simulink library "xrbsMath_r3"  (Simulink 5.0)
undefined symbols (not defined in the file or in its folder): num_width
libraries: xbsIndex_r3 x775, xrbsMath_r3 x16
(part 2 of 8)

== system xrbsMath_r3/CORDIC SQRT ==
  note: The CORDIC Square Root algorithm is implemented in 4 steps.
      |
      | Step 1: Co-ordinate Rotation.  The CORDIC algorithm converges only for positive values of x. If x < zero, the input data is
      | converted to a non-negative number. If x = 0, a zero detect flag is passed along. The Square Root circuit has been designed to
      | converge for all values of X, except for the most negative value .
      |
      | Step 2: Normalization.  The CORDIC algorithm converges only for 0.25 <= x < 1.0. During normalization, the input X is shifted to the
      | left till it has a 1 in the most significant bit after the signed bit. If the left shift resullted in an odd number of shift values, a right shift is
      | performed resulting in an even number of left shifts. The shift value is divided by 2 and passed on to the quadrant correct stage. The
      | square root is derived using the identity sqrt( w) = sqrt{ (w + 1/4)^2 - (w - 1/4)^2). Based on this identity the input w gets mapped to,
      | X = w + 0.25 and Y = w - 0.25.
      |
      | Step 3: Hyperbolic Rotations.  For sqrt(x^2 - y^2) calculation, the resulting vector is rotated through progressively smaller angles, such
      | that y goes to zero.
      |
      | Step 4: Co-ordinate Correction. If the input was negative and a left shift was applied to X, this step assigns the appropriate
      | sign to the resulting ratio and multiplies it with 2^(-shift). If the input was zero, the zero detect flag is used to set the output
      | to 0.
  x : Inport
  CORDIC Fine Angle PE : Subsystem  mask(CORDIC parallel PE){stages=stages, pe_nbits=norm_nbits+1, pe_binpt=norm_binpt, pipeline_x=pipeline, prev_stages=12, pipeline=[0  0  0  0  0  0  0  0  0  0  0  0]}
      mask prompts: stages "Number of Stages"; pe_nbits "Number of Bits"; pe_binpt "Binary Point Position"; pipeline_x "Pipeline Stage Value"; prev_stages "Previous Stages"; pipeline "Previous Pipeline Stage Value"
      mask init:
      | [bg,fg] = xlcmap('XBlock',0);
      | iPos = get_param(gcb,'Position');
      | iWidth=iPos(3)-iPos(1); iHeight=iPos(4)-iPos(2);
      | iCx=iWidth/2;
      | iCy=iHeight/2;
      | [logoX, logoY] = xlogo(iPos);
      | set_param(gcb,'LinkStatus', 'none');
      | sav_gcb=gcb;
      | stages = round(sum(abs(stages)));
      | if (stages == 0)
      | 	stages = prev_stages;
      | end
      | x = zeros(1,stages);
      | pipe_size = max(size(pipeline_x));
      | if pipe_size >= stages
      | 	x(1,1:stages) = pipeline_x(1,1:stages);
      | else
      | 	x(1,1:pipe_size) = pipeline_x(1,1:pipe_size);
      | end
      | 
      | if (stages ~=prev_stages)
      | 	pipeline = x;
      | 	a=find_system(sav_gcb, 'lookUnderMasks', 'all', 'FollowLinks','on','masktype', 'CORDIC iteration PE');
      | 	for i= 2:length(a)
      | 		for j=1:2
      | 		    delete_line(sav_gcb, ['CORDIC PE' int2str(i-1) '/' int2str(j)], ['CORDIC PE' int2str(i) '/' int2str(j)]);
      | 		end
      | 	end
      | 	delete_line(sav_gcb, ['CORDIC PE' int2str(length(a)) '/1'],'X/1');
      | 	delete_line(sav_gcb, ['CORDIC PE' int2str(length(a)) '/2'],'Terminator/1');
      | 	
      | 	for i=2:length(a)
      |       delete_block(a{i});
      | 	end
      | 	ite_stage=1;
      | 	repeat_stage=4;
      | 	dec_stage=0;
      | 	for i=2:stages
      |         ite_stage= i-dec_stage;
      | 		if(repeat_stage==ite_stage-1)
      |             ite_stage=ite_stage-1;
      | 			repeat_stage=repeat_stage*3+1;
      | 			dec_stage=dec_stage+1;
      | 		end
      |         add_block([sav_gcb '/CORDIC PE1'], [sav_gcb '/CORDIC PE' int2str(i)],'ii',int2str(ite_stage),'pipeline',['pipeline(1,' int2str(i) ')'],'position',[150+(i-1)*125, 70, 205+(i-1)*125, 130]);
      | 	end
      |     set_param([sav_gcb '/' 'X'], 'Position', [150+stages*125, 78, 180+stages*125, 92]);
      |     set_param([sav_gcb '/' 'Terminator'], 'Position', [210+stages*125, 107, 225+stages*125, 123]);
      |     for i= 2:stages
      | 		for j=1:2
      | 		    add_line(sav_gcb, ['CORDIC PE' int2str(i-1) '/' int2str(j)], ['CORDIC PE' int2str(i) '/' int2str(j)]);
      | 		end
      | 	end
      |     add_line(sav_gcb, ['CORDIC PE' int2str(stages) '/1'],'X/1');
      | 	add_line(sav_gcb, ['CORDIC PE' int2str(stages) '/2'],'Terminator/1');
      | 	find_system(sav_gcb, 'lookUnderMasks', 'all', 'FollowLinks', 'on', 'MaskType','Xilinx Slice Block');
      | 	set_param(sav_gcb, 'prev_stages',int2str(stages));
      | 	set_param(sav_gcb, 'pipeline', [ '[' int2str(x) ']']);
      | end
      | 
      | if (sum(pipeline~=x))
      | 	pipeline = x;
      | 	set_param(sav_gcb, 'pipeline', [ '[' int2str(x) ']']);
      | end
      mask Display:
      | patch([0 iWidth iWidth 0],[0 0 iHeight iHeight] , bg);
      | patch(logoX,logoY , fg);
      | port_label('input',1,'x');
      | port_label('input',2,'y');
      | port_label('input',3,'sgn(x)');
      | port_label('input',4,'shift');
      | port_label('input',5,'0_det');
      | port_label('output',1,'X');
      | port_label('output',2,'sgn(x)');
      | port_label('output',3,'shift');
      | port_label('output',4,'0_det');
      | plot([0 0 iWidth iWidth 0], [0 iHeight iHeight 0 0]);
  Quadrant Correct : Subsystem
      mask init:
      | [bg,fg] = xlcmap('XBlock',0);
      | iPos = get_param(gcb,'Position');
      | iWidth=iPos(3)-iPos(1); iHeight=iPos(4)-iPos(2);
      | iCx=iWidth/2;
      | iCy=iHeight/2;
      | [logoX, logoY] = xlogo(iPos);
      mask Display:
      | patch([0 iWidth iWidth 0],[0 0 iHeight iHeight] , bg);
      | patch(logoX,logoY , fg);
      | port_label('input',1,'X');
      | port_label('input',2,'sgn(x)');
      | port_label('input',3,'shift');
      | port_label('input',4,'0_det');
      | port_label('output',1,'X');
      | plot([0 0 iWidth iWidth 0], [0 iHeight iHeight 0 0]);
  Quadrant Map : Subsystem
      mask init:
      | [bg,fg] = xlcmap('XBlock',0);
      | iPos = get_param(gcb,'Position');
      | iWidth=iPos(3)-iPos(1); iHeight=iPos(4)-iPos(2);
      | iCx=iWidth/2;
      | iCy=iHeight/2;
      | [logoX, logoY] = xlogo(iPos);
      mask Display:
      | patch([0 iWidth iWidth 0],[0 0 iHeight iHeight] , bg);
      | patch(logoX,logoY , fg);
      | port_label('input',1,'x');
      | port_label('output',1,'X');
      | port_label('output',2,'Y');
      | port_label('output',3,'sgn(x)');
      | port_label('output',4,'shift');
      | port_label('output',5,'0_det');
      | plot([0 0 iWidth iWidth 0], [0 iHeight iHeight 0 0]);
  X : Outport
  wires:
  Quadrant Map/1(X) -> CORDIC Fine Angle PE/1(x)
  Quadrant Map/2(Y) -> CORDIC Fine Angle PE/2(y)
  Quadrant Correct/1(Z) -> X/1
  CORDIC Fine Angle PE/1(X) -> Quadrant Correct/1(X)
  x/1 -> Quadrant Map/1(x)
  Quadrant Map/3(sign(x)) -> CORDIC Fine Angle PE/3(sign)
  Quadrant Map/4(shift) -> CORDIC Fine Angle PE/4(shift)
  CORDIC Fine Angle PE/2(sign_dly) -> Quadrant Correct/2(sign_x)
  CORDIC Fine Angle PE/3(shift_dly) -> Quadrant Correct/3(shift)
  Quadrant Map/5(zero_detect) -> CORDIC Fine Angle PE/5(zero_detect)
  CORDIC Fine Angle PE/4(zero_detect_dly) -> Quadrant Correct/4(zero_detect)

== system xrbsMath_r3/CORDIC ATAN/CORDIC Fine Angle PE ==
  note: The fine angle rotation operation is performed iteratively in stages (0..stages-1).
      | The i-th PE rotates its input vector by an angle +/- atan(1/2^i), driving its input y coordinate towards zero.
  x : Inport
  y : Inport  Port=2
  z : Inport  Port=3
  CORDIC PE1 : Subsystem  mask(CORDIC iteration PE){ii=0, pe_nbits=pe_nbits, pe_binpt=pe_binpt, epsilon_k_fcn=atan, epsilon_k=, pipeline=pipeline(1,1)}
      mask prompts: ii "Iteration Index ii"; pe_nbits "Number of X,Y,Z Bits"; pe_binpt "X,Y,Z Binary Point Position"; epsilon_k_fcn "Epsilon_k Function"; pipeline "Pipeline Latency"
      mask init:
      | [bg,fg] = xlcmap('XBlock',0);
      | iPos = get_param(gcb,'Position');
      | iWidth=iPos(3)-iPos(1); iHeight=iPos(4)-iPos(2);
      | iCx=iWidth/2;
      | iCy=iHeight/2;
      | [logoX, logoY] = xlogo(iPos);
      | 
      | set_param(gcb, 'LinkStatus', 'none');
      | switch epsilon_k_fcn
      |   case 1
      |     epsilon_k = atan(1/2^ii);
      |   case 2
      |     epsilon_k = atanh(1/2^ii);
      | end
      mask StyleString: edit,edit,edit,popup(atan|atanh),edit,edit
      mask Display:
      | patch([0 iWidth iWidth 0],[0 0 iHeight iHeight] , bg);
      | patch(logoX,logoY , fg);
      | port_label('input',1,'x');
      | port_label('input',2,'y');
      | port_label('input',3,'z');
      | port_label('output',1,'X');
      | port_label('output',2,'Y');
      | port_label('output',3,'Z');
      | plot([0 0 iWidth iWidth 0], [0 iHeight iHeight 0 0]);
  CORDIC PE2 : Subsystem  mask(CORDIC iteration PE){ii=1, pe_nbits=pe_nbits, pe_binpt=pe_binpt, epsilon_k_fcn=atan, epsilon_k=, pipeline=pipeline(1,2)}
      mask prompts: ii "Iteration Index ii"; pe_nbits "Number of X,Y,Z Bits"; pe_binpt "X,Y,Z Binary Point Position"; epsilon_k_fcn "Epsilon_k Function"; pipeline "Pipeline Latency"
      mask init: same as xrbsMath_r3/CORDIC ATAN/CORDIC Fine Angle PE/CORDIC PE1
      mask StyleString: edit,edit,edit,popup(atan|atanh),edit,edit
      mask Display:
      | patch([0 iWidth iWidth 0],[0 0 iHeight iHeight] , bg);
      | patch(logoX,logoY , fg);
      | port_label('input',1,'x');
      | port_label('input',2,'y');
      | port_label('input',3,'z');
      | port_label('output',1,'X');
      | port_label('output',2,'Y');
      | port_label('output',3,'Z');
      | plot([0 0 iWidth iWidth 0], [0 iHeight iHeight 0 0]);
  CORDIC PE3 : Subsystem  mask(CORDIC iteration PE){ii=2, pe_nbits=pe_nbits, pe_binpt=pe_binpt, epsilon_k_fcn=atan, epsilon_k=, pipeline=pipeline(1,3)}
      mask prompts: ii "Iteration Index ii"; pe_nbits "Number of X,Y,Z Bits"; pe_binpt "X,Y,Z Binary Point Position"; epsilon_k_fcn "Epsilon_k Function"; pipeline "Pipeline Latency"
      mask init: same as xrbsMath_r3/CORDIC ATAN/CORDIC Fine Angle PE/CORDIC PE1
      mask StyleString: edit,edit,edit,popup(atan|atanh),edit,edit
      mask Display:
      | patch([0 iWidth iWidth 0],[0 0 iHeight iHeight] , bg);
      | patch(logoX,logoY , fg);
      | port_label('input',1,'x');
      | port_label('input',2,'y');
      | port_label('input',3,'z');
      | port_label('output',1,'X');
      | port_label('output',2,'Y');
      | port_label('output',3,'Z');
      | plot([0 0 iWidth iWidth 0], [0 iHeight iHeight 0 0]);
  CORDIC PE4 : Subsystem  mask(CORDIC iteration PE){ii=3, pe_nbits=pe_nbits, pe_binpt=pe_binpt, epsilon_k_fcn=atan, epsilon_k=, pipeline=pipeline(1,4)}
      mask prompts: ii "Iteration Index ii"; pe_nbits "Number of X,Y,Z Bits"; pe_binpt "X,Y,Z Binary Point Position"; epsilon_k_fcn "Epsilon_k Function"; pipeline "Pipeline Latency"
      mask init: same as xrbsMath_r3/CORDIC ATAN/CORDIC Fine Angle PE/CORDIC PE1
      mask StyleString: edit,edit,edit,popup(atan|atanh),edit,edit
      mask Display:
      | patch([0 iWidth iWidth 0],[0 0 iHeight iHeight] , bg);
      | patch(logoX,logoY , fg);
      | port_label('input',1,'x');
      | port_label('input',2,'y');
      | port_label('input',3,'z');
      | port_label('output',1,'X');
      | port_label('output',2,'Y');
      | port_label('output',3,'Z');
      | plot([0 0 iWidth iWidth 0], [0 iHeight iHeight 0 0]);
  CORDIC PE5 : Subsystem  mask(CORDIC iteration PE){ii=4, pe_nbits=pe_nbits, pe_binpt=pe_binpt, epsilon_k_fcn=atan, epsilon_k=, pipeline=pipeline(1,5)}
      mask prompts: ii "Iteration Index ii"; pe_nbits "Number of X,Y,Z Bits"; pe_binpt "X,Y,Z Binary Point Position"; epsilon_k_fcn "Epsilon_k Function"; pipeline "Pipeline Latency"
      mask init: same as xrbsMath_r3/CORDIC ATAN/CORDIC Fine Angle PE/CORDIC PE1
      mask StyleString: edit,edit,edit,popup(atan|atanh),edit,edit
      mask Display:
      | patch([0 iWidth iWidth 0],[0 0 iHeight iHeight] , bg);
      | patch(logoX,logoY , fg);
      | port_label('input',1,'x');
      | port_label('input',2,'y');
      | port_label('input',3,'z');
      | port_label('output',1,'X');
      | port_label('output',2,'Y');
      | port_label('output',3,'Z');
      | plot([0 0 iWidth iWidth 0], [0 iHeight iHeight 0 0]);
  CORDIC PE6 : Subsystem  mask(CORDIC iteration PE){ii=5, pe_nbits=pe_nbits, pe_binpt=pe_binpt, epsilon_k_fcn=atan, epsilon_k=, pipeline=pipeline(1,6)}
      mask prompts: ii "Iteration Index ii"; pe_nbits "Number of X,Y,Z Bits"; pe_binpt "X,Y,Z Binary Point Position"; epsilon_k_fcn "Epsilon_k Function"; pipeline "Pipeline Latency"
      mask init: same as xrbsMath_r3/CORDIC ATAN/CORDIC Fine Angle PE/CORDIC PE1
      mask StyleString: edit,edit,edit,popup(atan|atanh),edit,edit
      mask Display:
      | patch([0 iWidth iWidth 0],[0 0 iHeight iHeight] , bg);
      | patch(logoX,logoY , fg);
      | port_label('input',1,'x');
      | port_label('input',2,'y');
      | port_label('input',3,'z');
      | port_label('output',1,'X');
      | port_label('output',2,'Y');
      | port_label('output',3,'Z');
      | plot([0 0 iWidth iWidth 0], [0 iHeight iHeight 0 0]);
  CORDIC PE7 : Subsystem  mask(CORDIC iteration PE){ii=6, pe_nbits=pe_nbits, pe_binpt=pe_binpt, epsilon_k_fcn=atan, epsilon_k=, pipeline=pipeline(1,7)}
      mask prompts: ii "Iteration Index ii"; pe_nbits "Number of X,Y,Z Bits"; pe_binpt "X,Y,Z Binary Point Position"; epsilon_k_fcn "Epsilon_k Function"; pipeline "Pipeline Latency"
      mask init: same as xrbsMath_r3/CORDIC ATAN/CORDIC Fine Angle PE/CORDIC PE1
      mask StyleString: edit,edit,edit,popup(atan|atanh),edit,edit
      mask Display:
      | patch([0 iWidth iWidth 0],[0 0 iHeight iHeight] , bg);
      | patch(logoX,logoY , fg);
      | port_label('input',1,'x');
      | port_label('input',2,'y');
      | port_label('input',3,'z');
      | port_label('output',1,'X');
      | port_label('output',2,'Y');
      | port_label('output',3,'Z');
      | plot([0 0 iWidth iWidth 0], [0 iHeight iHeight 0 0]);
  CORDIC PE8 : Subsystem  mask(CORDIC iteration PE){ii=7, pe_nbits=pe_nbits, pe_binpt=pe_binpt, epsilon_k_fcn=atan, epsilon_k=, pipeline=pipeline(1,8)}
      mask prompts: ii "Iteration Index ii"; pe_nbits "Number of X,Y,Z Bits"; pe_binpt "X,Y,Z Binary Point Position"; epsilon_k_fcn "Epsilon_k Function"; pipeline "Pipeline Latency"
      mask init: same as xrbsMath_r3/CORDIC ATAN/CORDIC Fine Angle PE/CORDIC PE1
      mask StyleString: edit,edit,edit,popup(atan|atanh),edit,edit
      mask Display:
      | patch([0 iWidth iWidth 0],[0 0 iHeight iHeight] , bg);
      | patch(logoX,logoY , fg);
      | port_label('input',1,'x');
      | port_label('input',2,'y');
      | port_label('input',3,'z');
      | port_label('output',1,'X');
      | port_label('output',2,'Y');
      | port_label('output',3,'Z');
      | plot([0 0 iWidth iWidth 0], [0 iHeight iHeight 0 0]);
  Terminator : Terminator
  X : Outport
  Z : Outport  Port=2
  wires:
  CORDIC PE1/1(X) -> CORDIC PE2/1(x)
  CORDIC PE1/2(Y) -> CORDIC PE2/2(y)
  CORDIC PE1/3(Z) -> CORDIC PE2/3(z)
  CORDIC PE2/1(X) -> CORDIC PE3/1(x)
  CORDIC PE2/2(Y) -> CORDIC PE3/2(y)
  CORDIC PE2/3(Z) -> CORDIC PE3/3(z)
  CORDIC PE3/1(X) -> CORDIC PE4/1(x)
  CORDIC PE3/2(Y) -> CORDIC PE4/2(y)
  CORDIC PE3/3(Z) -> CORDIC PE4/3(z)
  CORDIC PE4/1(X) -> CORDIC PE5/1(x)
  CORDIC PE4/2(Y) -> CORDIC PE5/2(y)
  CORDIC PE4/3(Z) -> CORDIC PE5/3(z)
  CORDIC PE5/1(X) -> CORDIC PE6/1(x)
  CORDIC PE5/2(Y) -> CORDIC PE6/2(y)
  CORDIC PE5/3(Z) -> CORDIC PE6/3(z)
  CORDIC PE6/1(X) -> CORDIC PE7/1(x)
  CORDIC PE6/2(Y) -> CORDIC PE7/2(y)
  CORDIC PE6/3(Z) -> CORDIC PE7/3(z)
  CORDIC PE7/1(X) -> CORDIC PE8/1(x)
  CORDIC PE7/2(Y) -> CORDIC PE8/2(y)
  CORDIC PE7/3(Z) -> CORDIC PE8/3(z)
  x/1 -> CORDIC PE1/1(x)
  y/1 -> CORDIC PE1/2(y)
  z/1 -> CORDIC PE1/3(z)
  CORDIC PE8/1(X) -> X/1
  CORDIC PE8/2(Y) -> Terminator/1
  CORDIC PE8/3(Z) -> Z/1

== system xrbsMath_r3/CORDIC ATAN/Quadrant Correct ==
  note: The  CORDIC algorithm coverges for angles between  -pi/2 to +pi/2. The Quadrant Correct subsystem reflects
      | the angle back to the 2nd and 3rd quadrant from the 1st and 4th quadarnt if reflection was applied during the
      | quadarnt map stage. Reflection is applied by subtracting the output angle by pi if the original vector was in the
      | 2nd quadrant and -p if it was in the 3rd quadrant.
  Z IN : Inport
  PI_ addsub : Inport  Port=2
  Z MUX SEL : Inport  Port=3
  +PI : xbsIndex_r3/Constant  const=pi  arith_type="Signed  (2's comp)"  n_bits=pe_nbits  bin_pt=pe_binpt  explicit_period=off  period=1  dbl_ovrd=off
  -PI : xbsIndex_r3/Constant  const=-pi  arith_type="Signed  (2's comp)"  n_bits=pe_nbits  bin_pt=pe_binpt  explicit_period=off  period=1  dbl_ovrd=off
  AddSub : xbsIndex_r3/AddSub  mode=Subtraction  precision=User Defined  arith_type="Signed  (2's comp)"  n_bits=pe_nbits  bin_pt=pe_binpt  quantization=Truncate  overflow=Wrap  latency=0  explicit_period=off  period=1  en=off  dbl_ovrd=off  use_core=on  gen_core=on  pipeline=off  use_rpm=off
      settings: xl_area=[0, 0, 0, 0, 0, 0, 0]
  Convert : xbsIndex_r3/Convert  arith_type=Boolean  n_bits=8  bin_pt=6  quantization=Truncate  overflow=Wrap  latency=0  explicit_period=off  period=1  dbl_ovrd=off  inserted_by_tool=off
      settings: xl_area=[0, 0, 0, 0, 0, 0, 0]
  Mux : xbsIndex_r3/Mux  inputs=2  precision=Full  arith_type="Signed  (2's comp)"  n_bits=8  bin_pt=2  quantization=Truncate  overflow=Wrap  latency=1  mux_type=off  explicit_period=off  period=1  en=off  dbl_ovrd=off  gen_core=on  use_rpm=off
      settings: xl_area=[0, 0, 0, 0, 0, 0, 0]
  Mux1 : xbsIndex_r3/Mux  inputs=2  precision=Full  arith_type="Signed  (2's comp)"  n_bits=8  bin_pt=2  quantization=Truncate  overflow=Wrap  latency=0  mux_type=off  explicit_period=off  period=1  en=off  dbl_ovrd=off  gen_core=on  use_rpm=off
      settings: xl_area=[0, 0, 0, 0, 0, 0, 0]
  Z : Outport
  wires:
  -PI/1 -> Mux1/3
  +PI/1 -> Mux1/2
  Mux1/1 -> AddSub/1
  Convert/1 -> Mux1/1
  Z IN/1 -> Mux/2, AddSub/2
  Mux/1 -> Z/1
  AddSub/1 -> Mux/3
  Z MUX SEL/1 -> Mux/1
  PI_ addsub/1 -> Convert/1

== system xrbsMath_r3/CORDIC ATAN/Quadrant Map ==
  note: The  CORDIC algorithm converges for angles between  -pi/2 to +pi/2. The Quadrant Map subsystem always maps the
      | absolute value for x-axis. This reflects the input vector from the 2nd and 3rd quadrant to the 1st and 4th quadrant, resp.
  x : Inport
  y : Inport  Port=2
  Delay3 : xbsIndex_r3/Delay  latency=2  explicit_period=off  period=1  en=off  accept_only_valid=off  init_zero=on  dbl_ovrd=off
      settings: xl_area=[0, 0, 0, 0, 0, 0, 0]
  Delay4 : xbsIndex_r3/Delay  latency=1  explicit_period=off  period=1  en=off  accept_only_valid=off  init_zero=on  dbl_ovrd=off
      settings: xl_area=[0, 0, 0, 0, 0, 0, 0]
  Mux : xbsIndex_r3/Mux  inputs=2  precision=User Defined  arith_type="Signed  (2's comp)"  n_bits=pe_nbits  bin_pt=pe_binpt  quantization=Truncate  overflow=Wrap  latency=1  mux_type=off  explicit_period=off  period=1  en=off  dbl_ovrd=off  gen_core=on  use_rpm=off
      settings: xl_area=[0, 0, 0, 0, 0, 0, 0]
  Negate1 : xbsIndex_r3/Negate  precision=User Defined  arith_type="Signed  (2's comp)"  n_bits=pe_nbits  bin_pt=pe_binpt  quantization=Truncate  overflow=Wrap  latency=0  explicit_period=off  period=1  en=off  dbl_ovrd=off  use_core=on  gen_core=on  use_rpm=off
      settings: xl_area=[0, 0, 0, 0, 0, 0, 0]
  sgn(x) : xbsIndex_r3/Slice  mode=Upper Bit Location + Width  nbits=1  bit1=0  base1=MSB of Input  bit0=0  base0=LSB of Input  boolean_output=off  explicit_period=off  period=1  dbl_ovrd=off
  sgn(y) : xbsIndex_r3/Slice  mode=Upper Bit Location + Width  nbits=1  bit1=0  base1=MSB of Input  bit0=0  base0=LSB of Input  boolean_output=off  explicit_period=off  period=1  dbl_ovrd=off
  X : Outport
  Y : Outport  Port=2
  sign(y) : Outport  Port=3
  sign(x) : Outport  Port=4
  wires:
  Delay3/1 -> Y/1, sgn(y)/1
  Negate1/1 -> Mux/3
  Mux/1 -> X/1
  y/1 -> Delay3/1
  x/1 -> Delay4/1
  sgn(x)/1 -> Mux/1, sign(x)/1
  sgn(y)/1 -> sign(y)/1
  Delay4/1 -> sgn(x)/1, Negate1/1, Mux/2

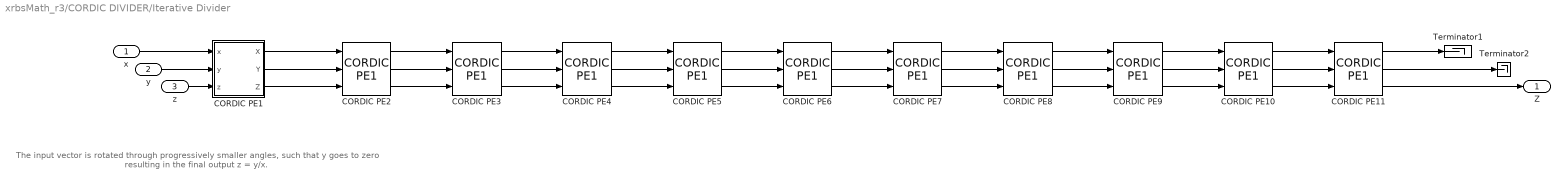
== system xrbsMath_r3/CORDIC DIVIDER/Iterative Divider ==
  note: The input vector is rotated through progressively smaller angles, such that y goes
      | to zero resulting in the final output z = y/x.
  x : Inport
  y : Inport  Port=2
  z : Inport  Port=3
  CORDIC PE1 : Subsystem  mask(CORDIC iteration Divider){ii=0, pe_nbits=num_width, pe_binpt=num_binpt, pipeline=pipeline(1,1), stages=stages}
      mask prompts: ii "Iteration Index ii"; pe_nbits "Number of X,Y,Z Bits"; pe_binpt "X,Y,Z Binary Point Position"; pipeline "Pipeline Latency"
      mask init:
      | [bg,fg] = xlcmap('XBlock',0);
      | iPos = get_param(gcb,'Position');
      | iWidth=iPos(3)-iPos(1); iHeight=iPos(4)-iPos(2);
      | iCx=iWidth/2;
      | iCy=iHeight/2;
      | [logoX, logoY] = xlogo(iPos);
      mask Display:
      | patch([0 iWidth iWidth 0],[0 0 iHeight iHeight] , bg);
      | patch(logoX,logoY , fg);
      | port_label('input',1,'x');
      | port_label('input',2,'y');
      | port_label('input',3,'z');
      | port_label('output',1,'X');
      | port_label('output',2,'Y');
      | port_label('output',3,'Z');
      | plot([0 0 iWidth iWidth 0], [0 iHeight iHeight 0 0]);
  CORDIC PE10 : xrbsMath_r3/CORDIC DIVIDER/Iterative Divider/CORDIC PE1  ii=9  pe_nbits=num_width  pe_binpt=num_binpt  pipeline=pipeline(1,10)  stages=stages
  CORDIC PE11 : xrbsMath_r3/CORDIC DIVIDER/Iterative Divider/CORDIC PE1  ii=10  pe_nbits=num_width  pe_binpt=num_binpt  pipeline=pipeline(1,11)  stages=stages
  CORDIC PE2 : xrbsMath_r3/CORDIC DIVIDER/Iterative Divider/CORDIC PE1  ii=1  pe_nbits=num_width  pe_binpt=num_binpt  pipeline=pipeline(1,2)  stages=stages
  CORDIC PE3 : xrbsMath_r3/CORDIC DIVIDER/Iterative Divider/CORDIC PE1  ii=2  pe_nbits=num_width  pe_binpt=num_binpt  pipeline=pipeline(1,3)  stages=stages
  CORDIC PE4 : xrbsMath_r3/CORDIC DIVIDER/Iterative Divider/CORDIC PE1  ii=3  pe_nbits=num_width  pe_binpt=num_binpt  pipeline=pipeline(1,4)  stages=stages
  CORDIC PE5 : xrbsMath_r3/CORDIC DIVIDER/Iterative Divider/CORDIC PE1  ii=4  pe_nbits=num_width  pe_binpt=num_binpt  pipeline=pipeline(1,5)  stages=stages
  CORDIC PE6 : xrbsMath_r3/CORDIC DIVIDER/Iterative Divider/CORDIC PE1  ii=5  pe_nbits=num_width  pe_binpt=num_binpt  pipeline=pipeline(1,6)  stages=stages
  CORDIC PE7 : xrbsMath_r3/CORDIC DIVIDER/Iterative Divider/CORDIC PE1  ii=6  pe_nbits=num_width  pe_binpt=num_binpt  pipeline=pipeline(1,7)  stages=stages
  CORDIC PE8 : xrbsMath_r3/CORDIC DIVIDER/Iterative Divider/CORDIC PE1  ii=7  pe_nbits=num_width  pe_binpt=num_binpt  pipeline=pipeline(1,8)  stages=stages
  CORDIC PE9 : xrbsMath_r3/CORDIC DIVIDER/Iterative Divider/CORDIC PE1  ii=8  pe_nbits=num_width  pe_binpt=num_binpt  pipeline=pipeline(1,9)  stages=stages
  Terminator1 : Terminator
  Terminator2 : Terminator
  Z : Outport
  wires:
  z/1 -> CORDIC PE1/3(z)
  y/1 -> CORDIC PE1/2(y)
  x/1 -> CORDIC PE1/1(x)
  CORDIC PE1/1(X) -> CORDIC PE2/1
  CORDIC PE1/2(Y) -> CORDIC PE2/2
  CORDIC PE1/3(Z) -> CORDIC PE2/3
  CORDIC PE2/1 -> CORDIC PE3/1
  CORDIC PE2/2 -> CORDIC PE3/2
  CORDIC PE2/3 -> CORDIC PE3/3
  CORDIC PE3/1 -> CORDIC PE4/1
  CORDIC PE3/2 -> CORDIC PE4/2
  CORDIC PE3/3 -> CORDIC PE4/3
  CORDIC PE4/1 -> CORDIC PE5/1
  CORDIC PE4/2 -> CORDIC PE5/2
  CORDIC PE4/3 -> CORDIC PE5/3
  CORDIC PE5/1 -> CORDIC PE6/1
  CORDIC PE5/2 -> CORDIC PE6/2
  CORDIC PE5/3 -> CORDIC PE6/3
  CORDIC PE6/1 -> CORDIC PE7/1
  CORDIC PE6/2 -> CORDIC PE7/2
  CORDIC PE6/3 -> CORDIC PE7/3
  CORDIC PE7/1 -> CORDIC PE8/1
  CORDIC PE7/2 -> CORDIC PE8/2
  CORDIC PE7/3 -> CORDIC PE8/3
  CORDIC PE8/1 -> CORDIC PE9/1
  CORDIC PE8/2 -> CORDIC PE9/2
  CORDIC PE8/3 -> CORDIC PE9/3
  CORDIC PE9/1 -> CORDIC PE10/1
  CORDIC PE9/2 -> CORDIC PE10/2
  CORDIC PE9/3 -> CORDIC PE10/3
  CORDIC PE10/1 -> CORDIC PE11/1
  CORDIC PE10/2 -> CORDIC PE11/2
  CORDIC PE10/3 -> CORDIC PE11/3
  CORDIC PE11/1 -> Terminator1/1
  CORDIC PE11/2 -> Terminator2/1
  CORDIC PE11/3 -> Z/1

== system xrbsMath_r3/CORDIC DIVIDER/Quadrant Correct ==
  note: Co-ordinate Correction. If the axis was rotated Step 1 and a relative shift was applied to Y over X, this step assigns the appropriate
      | sign to the resulting ratio and multiplies it with 2^(relative_shift of Y over X).
  z : Inport
  sign : Inport  Port=2
  norm : Inport  Port=3
  Mult : xbsIndex_r3/Mult  precision=Full  arith_type="Signed  (2's comp)"  n_bits=8  bin_pt=2  quantization=Truncate  overflow=Wrap  mult_type=Parallel  use_embedded=on  pipeline=on  latency=3  explicit_period=off  period=1  en=off  dbl_ovrd=off  oversample=2  use_rpm=off  placement_style=Rectangular Shape  gen_core=on
      settings: xl_area=[32 64 0 0 0 1 0]
  Mux : xbsIndex_r3/Mux  inputs=2  precision=Full  arith_type=Unsigned  n_bits=num_width-1  bin_pt=num_binpt  quantization=Truncate  overflow=Wrap  latency=0  mux_type=off  explicit_period=off  period=1  en=off  dbl_ovrd=off  use_rpm=off  gen_core=on
      settings: xl_area=[8 0 0 16 0 0 0]
  Negate : xbsIndex_r3/Negate  precision=User Defined  arith_type="Signed  (2's comp)"  n_bits=num_width  bin_pt=num_binpt  quantization=Truncate  overflow=Wrap  latency=0  explicit_period=off  period=1  en=off  dbl_ovrd=off  use_core=on  use_rpm=off  gen_core=on
      settings: xl_area=[8 0 0 16 0 0 0]
  ROM : xbsIndex_r3/ROM  depth=2^ceil(log2(num_width))  initVector=2.^(0:(2^ceil(log2(num_width))-1))  arith_type=Unsigned  n_bits=num_width  bin_pt=0  latency=0  distributed_mem=on  init_zero=on  explicit_period=off  period=1  rst=off  init_reg=0  en=off  dbl_ovrd=off  use_rpm=off  gen_core=on
      settings: xl_area=[8 0 0 16 0 0 0]
  Z : Outport
  wires:
  ROM/1 -> Mult/2
  Mult/1 -> Z/1
  norm/1 -> ROM/1
  Negate/1 -> Mux/3
  z/1 -> Negate/1, Mux/2
  sign/1 -> Mux/1
  Mux/1 -> Mult/1

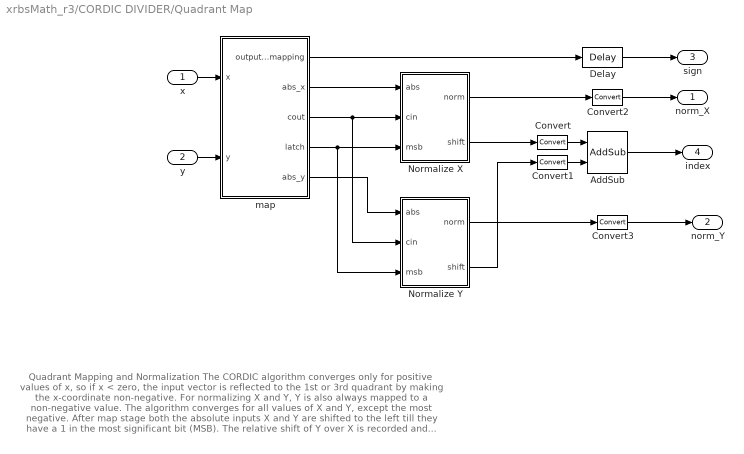
== system xrbsMath_r3/CORDIC DIVIDER/Quadrant Map ==
  note: Quadrant Mapping and Normalization
      |
      | The CORDIC algorithm converges only for positive values of x, so if x < zero, the input vector is reflected
      | to the 1st or 3rd quadrant by making the x-coordinate non-negative. For normalizing X and Y, Y is also
      | always mapped to a non-negative value. The algorithm converges for all values of X and Y, except the most negative.
      | After map stage both the absolute inputs X and Y are shifted to the left till they have a 1 in the most significant
      | bit (MSB). The relative shift of Y over X is recorded and passed on to the Quadrant Correct Stage.
  x : Inport
  y : Inport  Port=2
  AddSub : xbsIndex_r3/AddSub  mode=Subtraction  precision=User Defined  arith_type=Unsigned  n_bits=ceil(log2(num_width))  bin_pt=0  quantization=Truncate  overflow=Wrap  latency=0  explicit_period=off  period=1  en=off  dbl_ovrd=off  use_core=on  pipeline=off  use_rpm=off  gen_core=on
      settings: xl_area=[2 0 0 4 0 0 0]
  Convert : xbsIndex_r3/Convert  arith_type=Unsigned  n_bits=ceil(log2(num_width+1))  bin_pt=0  quantization=Truncate  overflow=Wrap  latency=0  explicit_period=off  period=1  dbl_ovrd=off  inserted_by_tool=off
      settings: xl_area=[0 0 0 0 0 0 0]
  Convert1 : xbsIndex_r3/Convert  arith_type=Unsigned  n_bits=ceil(log2(num_width+1))  bin_pt=0  quantization=Truncate  overflow=Wrap  latency=0  explicit_period=off  period=1  dbl_ovrd=off  inserted_by_tool=off
      settings: xl_area=[0 0 0 0 0 0 0]
  Convert2 : xbsIndex_r3/Convert  arith_type="Signed  (2's comp)"  n_bits=num_width  bin_pt=num_binpt  quantization=Truncate  overflow=Wrap  latency=0  explicit_period=off  period=1  dbl_ovrd=off  inserted_by_tool=off
      settings: xl_area=[0 0 0 0 0 0 0]
  Convert3 : xbsIndex_r3/Convert  arith_type="Signed  (2's comp)"  n_bits=num_width  bin_pt=num_binpt  quantization=Truncate  overflow=Wrap  latency=0  explicit_period=off  period=1  dbl_ovrd=off  inserted_by_tool=off
      settings: xl_area=[0 0 0 0 0 0 0]
  Delay : xbsIndex_r3/Delay  latency=num_width  reg_retiming=off  explicit_period=off  period=1  en=off  accept_only_valid=off  init_zero=on  dbl_ovrd=off
      settings: xl_area=[1 1 0 1 0 0 0]
  Normalize X : Subsystem  mask(Normalize X){num_bits=num_width-1, bin_point=num_binpt, prev_bits=15}
      mask prompts: num_bits "Number of bits"; bin_point "Binary Point Position"; prev_bits "Previous Number of bits"
      mask init:
      | [bg,fg] = xlcmap('XBlock',0);
      | iPos = get_param(gcb,'Position');
      | iWidth=iPos(3)-iPos(1); iHeight=iPos(4)-iPos(2);
      | iCx=iWidth/2;
      | iCy=iHeight/2;
      | [logoX, logoY] = xlogo(iPos);
      mask Display:
      | patch([0 iWidth iWidth 0],[0 0 iHeight iHeight] , bg);
      | patch(logoX,logoY , fg);
      | port_label('input',1,'abs');
      | port_label('input',2,'cin');
      | port_label('input',3,'msb');
      | port_label('output',1,'norm');
      | port_label('output',2,'shift');
      | plot([0 0 iWidth iWidth 0], [0 iHeight iHeight 0 0]);
  Normalize Y : Subsystem  mask(Normalize Y){num_bits=num_width-1, bin_point=num_binpt, prev_bits=15}
      mask prompts: num_bits "Number of bits"; bin_point "Binary Point Position"; prev_bits "Previous Number of bits"
      mask init:
      | [bg,fg] = xlcmap('XBlock',0);
      | iPos = get_param(gcb,'Position');
      | iWidth=iPos(3)-iPos(1); iHeight=iPos(4)-iPos(2);
      | iCx=iWidth/2;
      | iCy=iHeight/2;
      | [logoX, logoY] = xlogo(iPos);
      mask Display:
      | patch([0 iWidth iWidth 0],[0 0 iHeight iHeight] , bg);
      | patch(logoX,logoY , fg);
      | port_label('input',1,'abs');
      | port_label('input',2,'cin');
      | port_label('input',3,'msb');
      | port_label('output',1,'norm');
      | port_label('output',2,'shift');
      | plot([0 0 iWidth iWidth 0], [0 iHeight iHeight 0 0]);
  map : Subsystem
  norm_X : Outport
  norm_Y : Outport  Port=2
  sign : Outport  Port=3
  index : Outport  Port=4
  wires:
  map/1(output_mapping) -> Delay/1
  x/1 -> map/1(x)
  Normalize X/2(shift) -> Convert/1
  Normalize X/1(norm) -> Convert2/1
  Normalize Y/2(shift) -> Convert1/1
  Normalize Y/1(norm) -> Convert3/1
  y/1 -> map/2(y)
  map/2(abs_x) -> Normalize X/1(abs)
  map/3(cout) -> Normalize X/2(cin), Normalize Y/2(cin)
  map/4(latch) -> Normalize X/3(msb), Normalize Y/3(msb)
  map/5(abs_y) -> Normalize Y/1(abs)
  Convert/1 -> AddSub/1
  Convert1/1 -> AddSub/2
  AddSub/1 -> index/1
  Delay/1 -> sign/1
  Convert2/1 -> norm_X/1
  Convert3/1 -> norm_Y/1

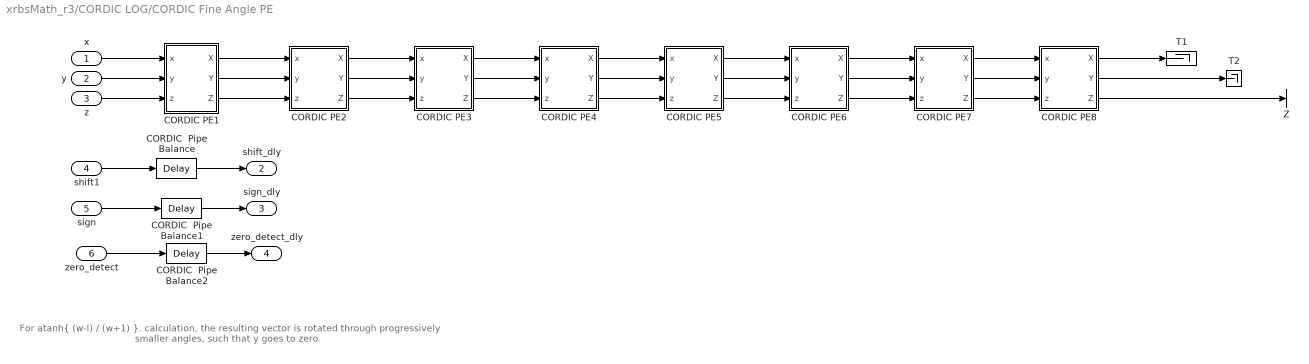
== system xrbsMath_r3/CORDIC LOG/CORDIC Fine Angle PE ==
  note: For atanh{ (w-l) / (w+1) }. calculation, the resulting vector is rotated through progressively smaller
      | angles, such that y goes to zero.
  x : Inport
  y : Inport  Port=2
  z : Inport  Port=3
  shift1 : Inport  Port=4
  sign : Inport  Port=5
  zero_detect : Inport  Port=6
  CORDIC  Pipe Balance : xbsIndex_r3/Delay  latency=sum(pipeline)  reg_retiming=off  explicit_period=off  period=1  en=off  accept_only_valid=off  init_zero=on  dbl_ovrd=off
      settings: xl_area=[1 1 0 1 0 0 0]
  CORDIC  Pipe Balance1 : xbsIndex_r3/Delay  latency=sum(pipeline)  reg_retiming=off  explicit_period=off  period=1  en=off  accept_only_valid=off  init_zero=on  dbl_ovrd=off
      settings: xl_area=[2 3 0 3 0 0 0]
  CORDIC  Pipe Balance2 : xbsIndex_r3/Delay  latency=sum(pipeline)  reg_retiming=off  explicit_period=off  period=1  en=off  accept_only_valid=off  init_zero=on  dbl_ovrd=off
      settings: xl_area=[1 1 0 1 0 0 0]
  CORDIC PE1 : Subsystem  mask(CORDIC iteration PE){ii=1, pe_nbits=pe_nbits, pe_binpt=pe_binpt, pipeline=pipeline(1,1)}
      mask prompts: ii "Iteration Index ii"; pe_nbits "Number of X,Y,Z Bits"; pe_binpt "X,Y,Z Binary Point Position"; pipeline "Pipeline Latency"
      mask init:
      | [bg,fg] = xlcmap('XBlock',0);
      | iPos = get_param(gcb,'Position');
      | iWidth=iPos(3)-iPos(1); iHeight=iPos(4)-iPos(2);
      | iCx=iWidth/2;
      | iCy=iHeight/2;
      | [logoX, logoY] = xlogo(iPos);
      | 
      | set_param(gcb, 'LinkStatus', 'none');
      mask Display:
      | patch([0 iWidth iWidth 0],[0 0 iHeight iHeight] , bg);
      | patch(logoX,logoY , fg);
      | port_label('input',1,'x');
      | port_label('input',2,'y');
      | port_label('input',3,'z');
      | port_label('output',1,'X');
      | port_label('output',2,'Y');
      | port_label('output',3,'Z');
      | plot([0 0 iWidth iWidth 0], [0 iHeight iHeight 0 0]);
  CORDIC PE2 : Subsystem  mask(CORDIC iteration PE){ii=2, pe_nbits=pe_nbits, pe_binpt=pe_binpt, pipeline=pipeline(1,2)}
      mask prompts: ii "Iteration Index ii"; pe_nbits "Number of X,Y,Z Bits"; pe_binpt "X,Y,Z Binary Point Position"; pipeline "Pipeline Latency"
      mask init: same as xrbsMath_r3/CORDIC LOG/CORDIC Fine Angle PE/CORDIC PE1
      mask Display:
      | patch([0 iWidth iWidth 0],[0 0 iHeight iHeight] , bg);
      | patch(logoX,logoY , fg);
      | port_label('input',1,'x');
      | port_label('input',2,'y');
      | port_label('input',3,'z');
      | port_label('output',1,'X');
      | port_label('output',2,'Y');
      | port_label('output',3,'Z');
      | plot([0 0 iWidth iWidth 0], [0 iHeight iHeight 0 0]);
  CORDIC PE3 : Subsystem  mask(CORDIC iteration PE){ii=3, pe_nbits=pe_nbits, pe_binpt=pe_binpt, pipeline=pipeline(1,3)}
      mask prompts: ii "Iteration Index ii"; pe_nbits "Number of X,Y,Z Bits"; pe_binpt "X,Y,Z Binary Point Position"; pipeline "Pipeline Latency"
      mask init: same as xrbsMath_r3/CORDIC LOG/CORDIC Fine Angle PE/CORDIC PE1
      mask Display:
      | patch([0 iWidth iWidth 0],[0 0 iHeight iHeight] , bg);
      | patch(logoX,logoY , fg);
      | port_label('input',1,'x');
      | port_label('input',2,'y');
      | port_label('input',3,'z');
      | port_label('output',1,'X');
      | port_label('output',2,'Y');
      | port_label('output',3,'Z');
      | plot([0 0 iWidth iWidth 0], [0 iHeight iHeight 0 0]);
  CORDIC PE4 : Subsystem  mask(CORDIC iteration PE){ii=4, pe_nbits=pe_nbits, pe_binpt=pe_binpt, pipeline=pipeline(1,4)}
      mask prompts: ii "Iteration Index ii"; pe_nbits "Number of X,Y,Z Bits"; pe_binpt "X,Y,Z Binary Point Position"; pipeline "Pipeline Latency"
      mask init: same as xrbsMath_r3/CORDIC LOG/CORDIC Fine Angle PE/CORDIC PE1
      mask Display:
      | patch([0 iWidth iWidth 0],[0 0 iHeight iHeight] , bg);
      | patch(logoX,logoY , fg);
      | port_label('input',1,'x');
      | port_label('input',2,'y');
      | port_label('input',3,'z');
      | port_label('output',1,'X');
      | port_label('output',2,'Y');
      | port_label('output',3,'Z');
      | plot([0 0 iWidth iWidth 0], [0 iHeight iHeight 0 0]);
  CORDIC PE5 : Subsystem  mask(CORDIC iteration PE){ii=4, pe_nbits=pe_nbits, pe_binpt=pe_binpt, pipeline=pipeline(1,5)}
      mask prompts: ii "Iteration Index ii"; pe_nbits "Number of X,Y,Z Bits"; pe_binpt "X,Y,Z Binary Point Position"; pipeline "Pipeline Latency"
      mask init: same as xrbsMath_r3/CORDIC LOG/CORDIC Fine Angle PE/CORDIC PE1
      mask Display:
      | patch([0 iWidth iWidth 0],[0 0 iHeight iHeight] , bg);
      | patch(logoX,logoY , fg);
      | port_label('input',1,'x');
      | port_label('input',2,'y');
      | port_label('input',3,'z');
      | port_label('output',1,'X');
      | port_label('output',2,'Y');
      | port_label('output',3,'Z');
      | plot([0 0 iWidth iWidth 0], [0 iHeight iHeight 0 0]);
  CORDIC PE6 : Subsystem  mask(CORDIC iteration PE){ii=5, pe_nbits=pe_nbits, pe_binpt=pe_binpt, pipeline=pipeline(1,6)}
      mask prompts: ii "Iteration Index ii"; pe_nbits "Number of X,Y,Z Bits"; pe_binpt "X,Y,Z Binary Point Position"; pipeline "Pipeline Latency"
      mask init: same as xrbsMath_r3/CORDIC LOG/CORDIC Fine Angle PE/CORDIC PE1
      mask Display:
      | patch([0 iWidth iWidth 0],[0 0 iHeight iHeight] , bg);
      | patch(logoX,logoY , fg);
      | port_label('input',1,'x');
      | port_label('input',2,'y');
      | port_label('input',3,'z');
      | port_label('output',1,'X');
      | port_label('output',2,'Y');
      | port_label('output',3,'Z');
      | plot([0 0 iWidth iWidth 0], [0 iHeight iHeight 0 0]);
  CORDIC PE7 : Subsystem  mask(CORDIC iteration PE){ii=6, pe_nbits=pe_nbits, pe_binpt=pe_binpt, pipeline=pipeline(1,7)}
      mask prompts: ii "Iteration Index ii"; pe_nbits "Number of X,Y,Z Bits"; pe_binpt "X,Y,Z Binary Point Position"; pipeline "Pipeline Latency"
      mask init: same as xrbsMath_r3/CORDIC LOG/CORDIC Fine Angle PE/CORDIC PE1
      mask Display:
      | patch([0 iWidth iWidth 0],[0 0 iHeight iHeight] , bg);
      | patch(logoX,logoY , fg);
      | port_label('input',1,'x');
      | port_label('input',2,'y');
      | port_label('input',3,'z');
      | port_label('output',1,'X');
      | port_label('output',2,'Y');
      | port_label('output',3,'Z');
      | plot([0 0 iWidth iWidth 0], [0 iHeight iHeight 0 0]);
  CORDIC PE8 : Subsystem  mask(CORDIC iteration PE){ii=7, pe_nbits=pe_nbits, pe_binpt=pe_binpt, pipeline=pipeline(1,8)}
      mask prompts: ii "Iteration Index ii"; pe_nbits "Number of X,Y,Z Bits"; pe_binpt "X,Y,Z Binary Point Position"; pipeline "Pipeline Latency"
      mask init: same as xrbsMath_r3/CORDIC LOG/CORDIC Fine Angle PE/CORDIC PE1
      mask Display:
      | patch([0 iWidth iWidth 0],[0 0 iHeight iHeight] , bg);
      | patch(logoX,logoY , fg);
      | port_label('input',1,'x');
      | port_label('input',2,'y');
      | port_label('input',3,'z');
      | port_label('output',1,'X');
      | port_label('output',2,'Y');
      | port_label('output',3,'Z');
      | plot([0 0 iWidth iWidth 0], [0 iHeight iHeight 0 0]);
  T1 : Terminator
  T2 : Terminator
  Z : Outport
  shift_dly : Outport  Port=2
  sign_dly : Outport  Port=3
  zero_detect_dly : Outport  Port=4
  wires:
  shift1/1 -> CORDIC  Pipe Balance/1
  CORDIC  Pipe Balance/1 -> shift_dly/1
  x/1 -> CORDIC PE1/1(x)
  y/1 -> CORDIC PE1/2(y)
  sign/1 -> CORDIC  Pipe Balance1/1
  CORDIC  Pipe Balance1/1 -> sign_dly/1
  zero_detect/1 -> CORDIC  Pipe Balance2/1
  CORDIC  Pipe Balance2/1 -> zero_detect_dly/1
  z/1 -> CORDIC PE1/3(z)
  CORDIC PE1/1(X) -> CORDIC PE2/1(x)
  CORDIC PE1/2(Y) -> CORDIC PE2/2(y)
  CORDIC PE1/3(Z) -> CORDIC PE2/3(z)
  CORDIC PE2/1(X) -> CORDIC PE3/1(x)
  CORDIC PE2/2(Y) -> CORDIC PE3/2(y)
  CORDIC PE2/3(Z) -> CORDIC PE3/3(z)
  CORDIC PE3/1(X) -> CORDIC PE4/1(x)
  CORDIC PE3/2(Y) -> CORDIC PE4/2(y)
  CORDIC PE3/3(Z) -> CORDIC PE4/3(z)
  CORDIC PE4/1(X) -> CORDIC PE5/1(x)
  CORDIC PE4/2(Y) -> CORDIC PE5/2(y)
  CORDIC PE4/3(Z) -> CORDIC PE5/3(z)
  CORDIC PE5/1(X) -> CORDIC PE6/1(x)
  CORDIC PE5/2(Y) -> CORDIC PE6/2(y)
  CORDIC PE5/3(Z) -> CORDIC PE6/3(z)
  CORDIC PE6/1(X) -> CORDIC PE7/1(x)
  CORDIC PE6/2(Y) -> CORDIC PE7/2(y)
  CORDIC PE6/3(Z) -> CORDIC PE7/3(z)
  CORDIC PE7/1(X) -> CORDIC PE8/1(x)
  CORDIC PE7/2(Y) -> CORDIC PE8/2(y)
  CORDIC PE7/3(Z) -> CORDIC PE8/3(z)
  CORDIC PE8/1(X) -> T1/1
  CORDIC PE8/2(Y) -> T2/1
  CORDIC PE8/3(Z) -> Z/1

== system xrbsMath_r3/CORDIC LOG/Quadrant Correct ==
  note: If the input was negative  a CMPLX_PI flag is porvided at the output for adding PI if a complex output is desired.
      | If a left shift was applied to X, this step adjusts the output by using the equation log (w * 2^E) = log (w) + E * log (2).
  X : Inport
  shift : Inport  Port=2
  sign_x : Inport  Port=3
  zero_detect : Inport  Port=4
  AddSub : xbsIndex_r3/AddSub  mode=Addition  precision=Full  arith_type=Unsigned  n_bits=8  bin_pt=0  quantization=Truncate  overflow=Wrap  latency=1  explicit_period=off  period=1  en=off  dbl_ovrd=off  use_core=on  pipeline=off  use_rpm=off  gen_core=off
      settings: xl_area=[2 0 0 4 0 0 0]
  AddSub1 : xbsIndex_r3/AddSub  mode=Subtraction  precision=Full  arith_type=Unsigned  n_bits=8  bin_pt=0  quantization=Truncate  overflow=Wrap  latency=0  explicit_period=off  period=1  en=off  dbl_ovrd=off  use_core=on  pipeline=off  use_rpm=off  gen_core=off
      settings: xl_area=[2 0 0 4 0 0 0]
  CMult : xbsIndex_r3/CMult  const=log(2)  const_n_bits=9  const_bin_pt=9  precision=Full  arith_type="Signed  (2's comp)"  n_bits=8  bin_pt=6  quantization="Round  (unbiased: +/- Inf)"  overflow=Wrap  mult_type=Parallel  mem_type=Distributed RAM  pipeline=off  latency=0  explicit_period=off  period=1  en=off  dbl_ovrd=off  oversample=2  use_rpm=off  placement_style=Rectangular Shape  gen_core=off
      settings: xl_area=[16 0 0 31 0 0 0]
  Constant1 : xbsIndex_r3/Constant  const=k_val  arith_type=Unsigned  n_bits=k_bits  bin_pt=0  explicit_period=off  period=1  dbl_ovrd=off
  Delay : xbsIndex_r3/Delay  latency=1  reg_retiming=off  explicit_period=off  period=1  en=off  accept_only_valid=off  init_zero=on  dbl_ovrd=off
      settings: xl_area=[0, 0, 0, 0, 0, 0, 0]
  Shift : xbsIndex_r3/Shift  shift_dir=Left  shift_bits=1  precision=Full  arith_type="Signed  (2's comp)"  n_bits=8  bin_pt=2  quantization=Truncate  overflow=Wrap  latency=0  explicit_period=off  period=1  en=off  dbl_ovrd=off
      settings: xl_area=[0, 0, 0, 0, 0, 0, 0]
  Terminator : Terminator
  Z : Outport
  CMPLX_PI : Outport  Port=2
  wires:
  Shift/1 -> AddSub/1
  Delay/1 -> CMPLX_PI/1
  zero_detect/1 -> Terminator/1
  sign_x/1 -> Delay/1
  shift/1 -> AddSub1/2
  Constant1/1 -> AddSub1/1
  AddSub1/1 -> CMult/1
  CMult/1 -> AddSub/2
  AddSub/1 -> Z/1
  X/1 -> Shift/1

== system xrbsMath_r3/CORDIC LOG/Quadrant Map ==
  note: The CORDIC algorithm converges only for positive values of x. If x < zero, the input data is converted to a non-negative number.
      |  If x = 0, a zero detect flag is passed along to the output stage. The Log circuit has been designed to converge for all values of X,
      | except for the most negative value .
      |
      | The CORDIC algorithm converges only for 0.5 <= x < 1.0. During normalization, the input X is shifted to the
      | left till it has a 1 in the most significant bit.The log output is derived using the identity log( w) = 2*atanh{ (w-l) / (w+1) }.
      | Based on this identity the input w gets mapped to, X = w + 1 and Y = w - 1.
  x : Inport
  Co-ordinate Correction : Subsystem
      mask Display:
      | patch([0 iWidth iWidth 0],[0 0 iHeight iHeight] , bg);
      | patch(logoX,logoY , fg);
      | port_label('input',1,'x');
      | port_label('output',1,'X');
      | port_label('output',2,'sgn(x)');
      | port_label('output',3,'0_det');
      | plot([0 0 iWidth iWidth 0], [0 iHeight iHeight 0 0]);
  Constant : xbsIndex_r3/Constant  const=0  arith_type=Unsigned  n_bits=1  bin_pt=0  explicit_period=off  period=1  dbl_ovrd=off
  Delay1 : xbsIndex_r3/Delay  latency=pe_nbits-1  reg_retiming=off  explicit_period=off  period=1  en=off  accept_only_valid=off  init_zero=on  dbl_ovrd=off
      settings: xl_area=[1 1 0 1 0 0 0]
  Delay2 : xbsIndex_r3/Delay  latency=pe_nbits-1  reg_retiming=off  explicit_period=off  period=1  en=off  accept_only_valid=off  init_zero=on  dbl_ovrd=off
      settings: xl_area=[1 1 0 1 0 0 0]
  Normalize X : Subsystem  mask(Normalization Stage){num_bits=pe_nbits, bin_point=pe_nbits-1, prev_stages=7}
      mask prompts: num_bits "Number of bits"; bin_point "Binary Point Position"; prev_stages "Previous Number of bits"
      mask init:
      | [bg,fg] = xlcmap('XBlock',0);
      | iPos = get_param(gcb,'Position');
      | iWidth=iPos(3)-iPos(1); iHeight=iPos(4)-iPos(2);
      | iCx=iWidth/2;
      | iCy=iHeight/2;
      | [logoX, logoY] = xlogo(iPos);
      | set_param(gcb,'LinkStatus', 'none');
      | sav_gcb=gcb;
      | stages = round(sum(abs(num_bits-1)));
      | if (stages == 0)
      | 	stages = prev_stages;
      | end
      | if (stages ~=prev_stages)
      | 	a=find_system(gcb, 'lookUnderMasks', 'all', 'FollowLinks','on','masktype', 'Normalize Shift Stage');
      | 	for i= 2:length(a)
      | 		for j=1:3
      | 		    delete_line(sav_gcb, ['Shift' int2str(i-1) '/' int2str(j)], ['Shift' int2str(i) '/' int2str(j)]);
      | 		end
      | 	end
      | 	delete_line(sav_gcb, ['Shift' int2str(length(a)) '/1'],'norm/1');
      | 	delete_line(sav_gcb, ['Shift' int2str(length(a)) '/2'],'shift/1');
      | 	delete_line(sav_gcb, ['Shift' int2str(length(a)) '/3'],'Terminator1/1');
      | 	
      | 	for i=2:length(a)
      |       delete_block(a{i});
      | 	end
      | 	for i=2:stages,
      |         add_block([sav_gcb '/Shift1'], [sav_gcb '/Shift' int2str(i)],'position',[150+(i-1)*125, 70, 205+(i-1)*125, 130]);
      | 	end
      |     set_param([sav_gcb '/' 'norm'], 'Position', [150+stages*125, 72, 180+stages*125, 86]);
      |     set_param([sav_gcb '/' 'shift'], 'Position', [210+stages*125, 92, 225+stages*125, 108]);
      |     set_param([sav_gcb '/' 'Terminator1'], 'Position', [240+stages*125, 113, 270+stages*125, 127]);
      |     for i= 2:stages
      | 		for j=1:3
      | 		    add_line(sav_gcb, ['Shift' int2str(i-1) '/' int2str(j)], ['Shift' int2str(i) '/' int2str(j)]);
      | 		end
      | 	end
      |     add_line(sav_gcb, ['Shift' int2str(stages) '/1'],'norm/1');
      | 	add_line(sav_gcb, ['Shift' int2str(stages) '/2'],'shift/1');
      | 	add_line(sav_gcb, ['Shift' int2str(stages) '/3'],'Terminator1/1');
      | 	find_system(sav_gcb, 'lookUnderMasks', 'all', 'FollowLinks', 'on', 'MaskType','Xilinx Multiplexer Block');
      | 	set_param(sav_gcb, 'prev_stages',int2str(stages));
      | end
      mask Display:
      | patch([0 iWidth iWidth 0],[0 0 iHeight iHeight] , bg);
      | patch(logoX,logoY , fg);
      | port_label('input',1,'abs');
      | port_label('input',2,'cin');
      | port_label('input',3,'msb');
      | port_label('output',1,'norm');
      | port_label('output',2,'shift');
      | plot([0 0 iWidth iWidth 0], [0 iHeight iHeight 0 0]);
  Post Normalization : Subsystem
      mask Display:
      | patch([0 iWidth iWidth 0],[0 0 iHeight iHeight] , bg);
      | patch(logoX,logoY , fg);
      | port_label('input',1,'norm_x');
      | port_label('input',2,'shift');
      | port_label('output',1,'X');
      | port_label('output',2,'Y');
      | port_label('output',3,'Z');
      | port_label('output',4,'shift');
      | plot([0 0 iWidth iWidth 0], [0 iHeight iHeight 0 0]);
  X : Outport
  Y : Outport  Port=2
  shift : Outport  Port=3
  shift1 : Outport  Port=4
  sign : Outport  Port=5
  zero_detect : Outport  Port=6
  wires:
  Delay1/1 -> sign/1
  Co-ordinate Correction/2(sign_x) -> Delay1/1
  Post Normalization/4(shift_out) -> shift1/1
  Post Normalization/2(Y) -> Y/1
  Post Normalization/1(X) -> X/1
  Normalize X/2(shift) -> Post Normalization/2(shift_in)
  Normalize X/1(norm) -> Post Normalization/1(norm_x)
  Delay2/1 -> zero_detect/1
  Co-ordinate Correction/3(zero_detect) -> Delay2/1
  Post Normalization/3(Z) -> shift/1
  Constant/1 -> Normalize X/3(msb), Normalize X/2(cin)
  Co-ordinate Correction/1(X) -> Normalize X/1(abs)
  x/1 -> Co-ordinate Correction/1(x)
